simulink model "DoD_simulink_model"  (R2018b)
settings: Solver=FixedStepAuto  StartTime=0.0  StopTime=tsim  FixedStep=T  RelTol=1e-3
values from neighbouring files (symbols this model uses):
  a1 = 4.2005e3    (= 4200.5)    [DoD_simulation.m]    (also in Hamiltonian_sim.m = 6.5035)
  a2 = 0.0872    [DoD_simulation.m]    (also in Hamiltonian_sim.m = 0.00063853)
  a3 = 6.0509e-4    (= 0.00060509)    [DoD_simulation.m]    (also in Hamiltonian_sim.m = 0.0011)
  a4 = 1.8451    [DoD_simulation.m]    (also in Hamiltonian_sim.m = 0.025)
  a5 = 0.3583    [DoD_simulation.m]    (also in Hamiltonian_sim.m = 0.1042)
  a6 = 2.8311e-4    (= 0.00028311)    [DoD_simulation.m]    (also in Hamiltonian_sim.m = 0.0012)
  B1 = 1.0011e3    (= 1001.1)    [DoD_simulation.m]    (also in Hamiltonian_sim.m = 3002.1)
  B2 = 1.0023e3    (= 1002.3)    [DoD_simulation.m]    (also in Hamiltonian_sim.m = 986.7121)
  B3 = 7.9317e4    (= 79317)    [DoD_simulation.m]    (also in Hamiltonian_sim.m = 210000)
  B4 = 2.2251e5    (= 222510)    [DoD_simulation.m]    (also in Hamiltonian_sim.m = 19998)
  B5 = 1.5441e4    (= 15441)    [DoD_simulation.m]    (also in Hamiltonian_sim.m = 35000)
  B6 = 3.2077e4    (= 32077)    [DoD_simulation.m]    (also in Hamiltonian_sim.m = 19998)
  Cm = [0, 0, 1, 0 ... (first row only)    [DoD_simulation.m]    (also in Hamiltonian_sim.m = [1, 0, 0, 0)
  DD = [0.00, 0; 0, 0]    [DoD_simulation.m]
  Dm = [0;0]    [DoD_simulation.m]    (also in Hamiltonian_sim.m = [0; 0; 0])
  g = 9.82    [DoD_simulation.m]    (also in Hamiltonian_sim.m)
  Kc = zeros(1,length(idx))    [DoD_simulation.m]    (also in Hamiltonian_sim.m)
  Kw = 0.0086    [DoD_simulation.m]    (also in Hamiltonian_sim.m)
  MM = [ ... (first row only)    [DoD_simulation.m]
  mo = pi*(ro^2)*thick*p    (= 0.135716802635)    [DoD_simulation.m]    (also in Hamiltonian_sim.m)
  mup_init = [0; 0; theta0; phi0]    [DoD_simulation.m]    (also in Hamiltonian_sim.m)
  N = 98.78    [DoD_simulation.m]    (also in Hamiltonian_sim.m)
  Nu = NN(end)    [DoD_simulation.m]    (also in Hamiltonian_sim.m)
  Nx = zeros(length(Cr),1)    [DoD_simulation.m]    (also in Hamiltonian_sim.m)
  p1 = 0.7427    [DoD_simulation.m]    (also in Hamiltonian_sim.m = -4 + 0.5i)
  p2 = -0.2106    [DoD_simulation.m]    (also in Hamiltonian_sim.m = -4 - 0.5i)
  p3 = 1.121    [DoD_simulation.m]    (also in Hamiltonian_sim.m = -1.9)
  phi0 = -0*(pi/180)    (= 0)    [DoD_simulation.m]    (also in Hamiltonian_sim.m = 0.0174532925199)
  Pp_init = diag([0.1, 0.1, 0.1, 0.1])    [DoD_simulation.m]    (also in Hamiltonian_sim.m = diag([1e0, 1e0, 1e0, 1e0]))
  Qo = 0.001*eye(size(A,1))    [DoD_simulation.m]    (also in Hamiltonian_sim.m = diag([1e-10, 1e-10, 1e-10, 1e-10]))
  Ra = 2.5625    [DoD_simulation.m]    (also in Hamiltonian_sim.m)
  rh = 0.12    [DoD_simulation.m]    (also in Hamiltonian_sim.m)
  Ro = 0.001*eye(size(Cm,1))    [DoD_simulation.m]    (also in Hamiltonian_sim.m = diag([1e3, 1e3, 1e3]))
  ro = 0.06    [DoD_simulation.m]    (also in Hamiltonian_sim.m)
  theta0 = 0*(pi/180)    (= 0)    [DoD_simulation.m]    (also in Hamiltonian_sim.m)
undefined symbols (not defined in the file or in its folder): Aod, Bod
settings Model: Creator=timot  LastModifiedBy=Tim
settings DebuggingCC: AlgebraicLoopMsg=none  LibraryContextMissingDiagnostic=none
settings SFSimCC: SimUseLocalCustomCode=off
settings RTWCC: RTWUseLocalCustomCode=off

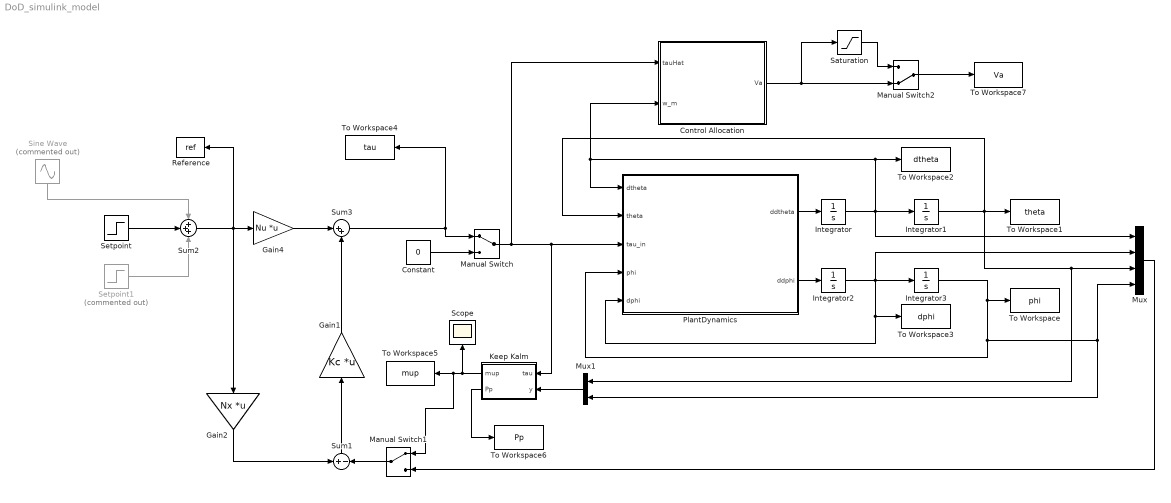
== system DoD_simulink_model ==
  Constant : Constant  Value=0
  Control Allocation : MATLAB Function  TreatAsAtomicUnit=on
  Gain1 : Gain  Gain=Kc  Multiplication=Matrix(K*u)
  Gain2 : Gain  Gain=Nx  Multiplication=Matrix(K*u)
  Gain4 : Gain  Gain=Nu  Multiplication=Matrix(K*u)
  Integrator : Integrator
  Integrator1 : Integrator  InitialCondition=theta0
  Integrator2 : Integrator
  Integrator3 : Integrator  InitialCondition=phi0
  Keep Kalm : Subsystem
  Manual Switch : ManualSwitch
  Manual Switch1 : ManualSwitch
  Manual Switch2 : ManualSwitch  CurrentSetting=0
  Mux : Mux
  Mux1 : Mux  Inputs=2
  "PlantDynamics " : MATLAB Function  TreatAsAtomicUnit=on
  Reference : ToWorkspace  VariableName=ref  SaveFormat=Structure With Time  SampleTime=-1
  Saturation : Saturate  UpperLimit=6  LowerLimit=-6
  Scope : Scope
  Setpoint : Step  Time=3  After=pi  SampleTime=0
  Setpoint1 : Step  Commented=on  Time=6  After=-pi  SampleTime=0
  Sine Wave : Sin  Commented=on  Amplitude=3  SampleTime=0
  Sum1 : Sum  Inputs=+|-
  Sum2 : Sum  Inputs=+++
  Sum3 : Sum  Inputs=|++
  To Workspace : ToWorkspace  VariableName=phi  SaveFormat=Structure With Time  SampleTime=-1
  To Workspace1 : ToWorkspace  VariableName=theta  SaveFormat=Structure With Time  SampleTime=-1
  To Workspace2 : ToWorkspace  VariableName=dtheta  SaveFormat=Structure With Time  SampleTime=-1
  To Workspace3 : ToWorkspace  VariableName=dphi  SaveFormat=Structure With Time  SampleTime=-1
  To Workspace4 : ToWorkspace  VariableName=tau  SaveFormat=Structure With Time  SampleTime=-1
  To Workspace5 : ToWorkspace  VariableName=mup  SaveFormat=Structure With Time  SampleTime=-1
  To Workspace6 : ToWorkspace  VariableName=Pp  SaveFormat=Structure With Time  SampleTime=-1
  To Workspace7 : ToWorkspace  VariableName=Va  SaveFormat=Structure With Time  SampleTime=-1
  wires:
  "PlantDynamics "/1(ddtheta) -> Integrator/1
  Integrator/1 -> Integrator1/1, Mux/1, "PlantDynamics "/1(dtheta), Control Allocation/2(w_m), To Workspace2/1
  "PlantDynamics "/2(ddphi) -> Integrator2/1
  Integrator2/1 -> Mux/2, "PlantDynamics "/5(dphi), To Workspace3/1, Integrator3/1
  Integrator1/1 -> Mux1/1, Mux/3, "PlantDynamics "/2(theta), To Workspace1/1
  Integrator3/1 -> Mux1/2, Mux/4, "PlantDynamics "/4(phi), To Workspace/1
  Gain4/1 -> Sum3/1
  Sum2/1 -> Gain4/1, Gain2/1, Reference/1
  Sum1/1 -> Gain1/1
  Gain2/1 -> Sum1/1
  Gain1/1 -> Sum3/2
  Sum3/1 -> To Workspace4/1, Manual Switch/1
  Constant/1 -> Manual Switch/2
  Manual Switch/1 -> Control Allocation/1(tauHat), "PlantDynamics "/3(tau_in), Keep Kalm/1(tau)
  Manual Switch1/1 -> Sum1/2
  Mux/1 -> Manual Switch1/2
  Keep Kalm/1(mup) -> Manual Switch1/1, To Workspace5/1, Scope/1
  Keep Kalm/2(Pp) -> To Workspace6/1
  Mux1/1 -> Keep Kalm/2(y)
  Control Allocation/1(Va) -> Manual Switch2/2, Saturation/1
  Setpoint/1 -> Sum2/2
  Setpoint1/1 -> Sum2/3
  Sine Wave/1 -> Sum2/1
  Manual Switch2/1 -> To Workspace7/1
  Saturation/1 -> Manual Switch2/1

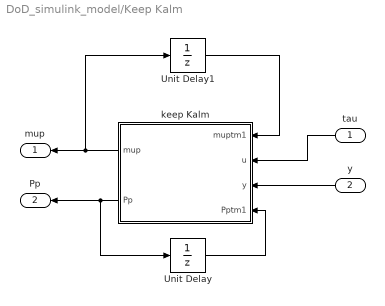
== system DoD_simulink_model/Keep Kalm ==
  tau : Inport
  y : Inport  Port=2
  Unit Delay : UnitDelay  InitialCondition=Pp_init  SampleTime=-1
  Unit Delay1 : UnitDelay  InitialCondition=mup_init  SampleTime=-1
  "keep Kalm " : MATLAB Function  TreatAsAtomicUnit=on
  mup : Outport
  Pp : Outport  Port=2
  wires:
  "keep Kalm "/2(Pp) -> Unit Delay/1, Pp/1
  tau/1 -> "keep Kalm "/2(u)
  "keep Kalm "/1(mup) -> Unit Delay1/1, mup/1
  Unit Delay/1 -> "keep Kalm "/4(Pptm1)
  Unit Delay1/1 -> "keep Kalm "/1(muptm1)
  y/1 -> "keep Kalm "/3(y)

== matlab function DoD_simulink_model/Keep Kalm/keep Kalm  ==
  data: muptm1 input; u input; y input; Pptm1 input; Cm parameter; Bod parameter; Qo parameter; Ro parameter; Aod parameter; Dm parameter; mup output; Pp output
function [mup, Pp] = fcn(muptm1, u, y,  Pptm1, Cm, Bod, Qo, Ro, Aod, Dm)

% Update with new measurement
muf = muptm1 + Pptm1*Cm'*((Cm*Pptm1*Cm' + Ro)\(y - Cm*muptm1 - Dm*u));
Pf = Pptm1 - Pptm1*Cm'*((Cm*Pptm1*Cm' + Ro)\(Cm*Pptm1));

% Predict Forward
mup = Aod*muf + Bod*u;
Pp = Aod*Pf*Aod' + Qo;


% muf = mup(:,t) + Pp(:,:,t)*C'*((C*Pp(:,:,t)*C' + R)\(mup(:,t) - C*mup(:,t) - D*u(:,t)));
% Pf(:,:,t) = Pp(:,:,t) - Pp(:,:,t)*C'*((C*Pp(:,:,t)*C' + R)\(C*Pp(:,:,t)));
% %Predict forward
% mup(:,t+1) = A*muf(:,t) + B*u(:,t);
% Pp(:,:,t+1) = A*Pf(:,:,t)*A' + Q;
% 
%

== matlab function DoD_simulink_model/PlantDynamics  ==
  data: dtheta input; theta input; tau_in input; ddtheta output; ddphi output; MM parameter; phi input; dphi input; mo parameter; ro parameter; rh parameter; g parameter; DD parameter
function [ddtheta, ddphi] = DoDPlantModel(dtheta, theta, tau_in, MM, phi, dphi, mo, ro, rh, g, DD)


qdot = [dtheta; dphi];

gq = [0; -mo*g*(rh + ro)*sin(phi)];

tau_in = [tau_in; 0];
out = MM\(tau_in - DD*qdot - gq);
% out = MM\(tau_in - gq);
ddtheta = out(1);
ddphi = out(2);

== matlab function DoD_simulink_model/Control Allocation ==
  data: tauHat input; Va output; w_m input; Ra parameter; Kw parameter; N parameter; a1 parameter; a2 parameter; a3 parameter; B1 parameter; B2 parameter; B3 parameter; a4 parameter; a5 parameter; a6 parameter; B4 parameter; B5 parameter; B6 parameter; p1 parameter; p2 parameter; p3 parameter
function Va = controlAllocation(tauHat, w_m, Ra, Kw, N, a1, a2, a3, B1, B2,...
    B3, a4, a5, a6, B4, B5, B6, p1, p2, p3)
% Correct velocity
w_m = w_m.*N;

% Heaviside functions
heavi_p =@(x) 1./(1 + exp(-2.*50.*x));
heavi_m =@(x) 1./(1 + exp(-2.*50.*-x));

% Friction function
tauF = (a1.*(tanh(B1.*w_m) - tanh(B2.*w_m)) + a2.*tanh(B3.*w_m) + a3.*w_m).*heavi_p(w_m)...
                + (a4.*(tanh(B4.*w_m) - tanh(B5.*w_m)) + a5.*tanh(B6.*w_m) + a6.*w_m).*heavi_m(w_m);

% Motor torque
Tm = tauHat + tauF;

% Current
Ia =  p1.*Tm.^3 + p2.*Tm.^2 + p3.*Tm;

% Voltage
Va = Kw.*w_m + Ra.*Ia;
